simulink model "mm_autograde_M1b_nice"  (R2025a)
settings: Solver=FixedStepAuto  StartTime=0.0  StopTime=30  FixedStep=0.005  RelTol=1e-3
libraries: mmuct_lib x2
settings Model: PacingRate=2  Creator=nicolls  LastModifiedBy=llamalulu
settings RTWCC: GenCodeOnly=on

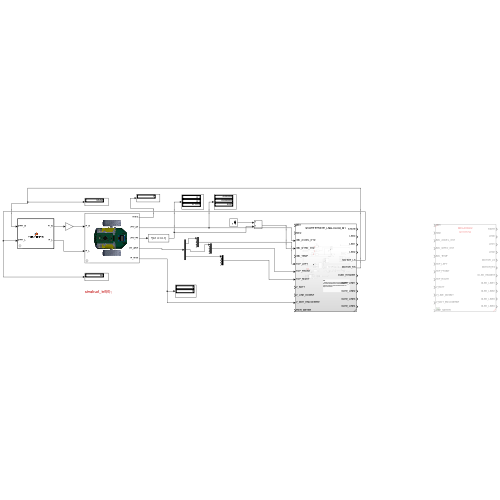
[thumbnail: Simulink's stored preview of the top-level diagram]
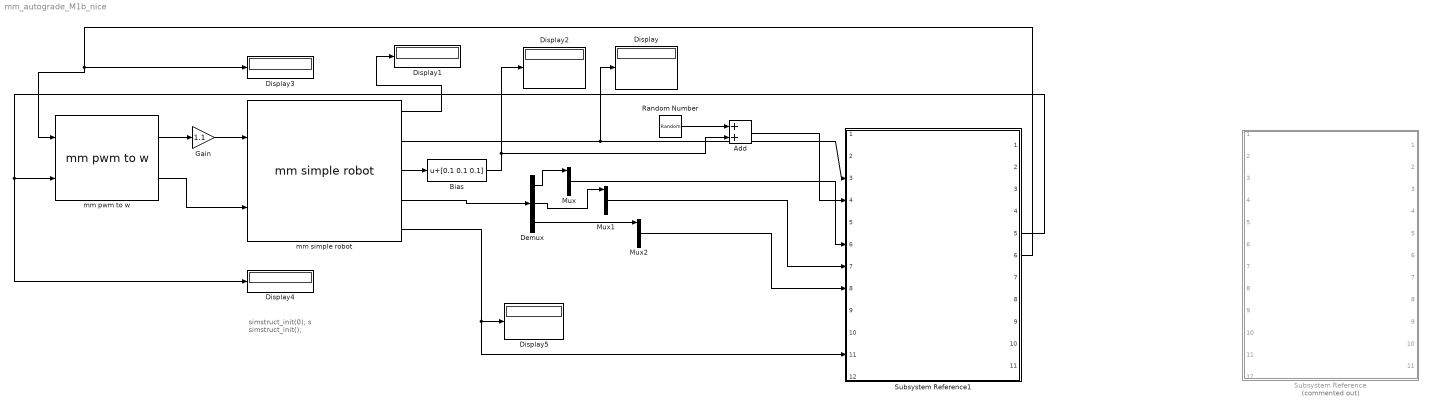
== system mm_autograde_M1b_nice ==
  note: simstruct_init(0);
      | s
      | simstruct_init();
  Add : Sum
  Bias : Bias  Bias=[0.1 0.1 0.1]  SaturateOnIntegerOverflow=off
  Demux : Demux  Outputs=3
  Display{,1..5} (6 alike) : Display
  Gain : Gain  Gain=1.1
  Mux : Mux
  Mux1 : Mux
  Mux2 : Mux
  Random Number : RandomNumber  Variance=0.05  SampleTime=0.1
  Subsystem Reference : Subsystem  Commented=on  ReferencedSubsystem=MDLAYA022
  Subsystem Reference1 : Subsystem  ReferencedSubsystem=StudentTemplate_LNGLUL002_M1
  mm pwm to w : mmuct_lib/mm pwm to w  deadb=0  maxw=2*pi  motd=0
  mm simple robot : mmuct_lib/mm simple robot  simstruct=simstruct  x0=0.3  y0=0.75  theta0=0
      settings: SourceProductName=UCT EEE Micromouse
  wires:
  Demux/1 -> Mux/1
  Demux/2 -> Mux1/1
  Demux/3 -> Mux2/1
  Subsystem Reference1/6 -> Display3/1, mm pwm to w/1
  mm simple robot/3 -> Bias/1
  mm simple robot/1 -> Display1/1
  mm simple robot/5 -> Subsystem Reference1/11, Display5/1
  mm pwm to w/2 -> mm simple robot/2
  mm pwm to w/1 -> Gain/1
  Mux2/1 -> Subsystem Reference1/8
  Mux1/1 -> Subsystem Reference1/7
  Mux/1 -> Subsystem Reference1/6
  mm simple robot/2 -> Subsystem Reference1/3, Display/1
  Subsystem Reference1/5 -> mm pwm to w/2, Display4/1
  mm simple robot/4 -> Demux/1
  Gain/1 -> mm simple robot/1
  Bias/1 -> Add/2, Display2/1
  Random Number/1 -> Add/1
  Add/1 -> Subsystem Reference1/4
